simulink model "hard_threshold_fixed_multichannel"  (R2019b)
settings: Solver=VariableStepAuto  StartTime=0.0  StopTime=10  RelTol=1e-3
libraries: simulink x33, dspswit3 x1
settings Model: Creator=sbuccelli  LastModifiedBy=sbuccelli

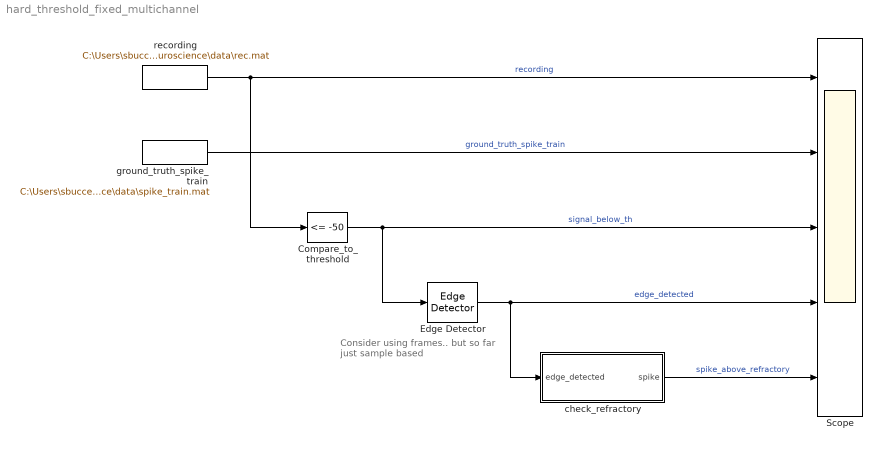
== system hard_threshold_fixed_multichannel ==
  note: Consider using frames..
      | but so far just sample based
  Compare_to_threshold : simulink/Logic and Bit Operations/Compare To Constant  relop=<=  const=-50  OutDataTypeStr=boolean
  Edge Detector : dspswit3/Edge Detector
      settings: SourceProductName=DSP System Toolbox  SourceProductBaseCode=DS
  Scope : Scope  NumInputPorts=5
  check_refractory : Subsystem
  ground_truth_spike_train : FromFile  FileName=C:\Users\sbuccelli\Documents\GitHub\closed-loop-neuroscience\data\spike_train.mat  SampleTime=1/32e3
  recording : FromFile  FileName=C:\Users\sbuccelli\Documents\GitHub\closed-loop-neuroscience\data\rec.mat  SampleTime=1/32e3
  wires:
  recording/1 -> Compare_to_threshold/1, Scope/1  "recording"
  ground_truth_spike_train/1 -> Scope/2  "ground_truth_spike_train"
  Compare_to_threshold/1 -> Edge Detector/1, Scope/3  "signal_below_th"
  Edge Detector/1 -> check_refractory/1(edge_detected), Scope/4  "edge_detected"
  check_refractory/1(spike) -> Scope/5  "spike_above_refractory"

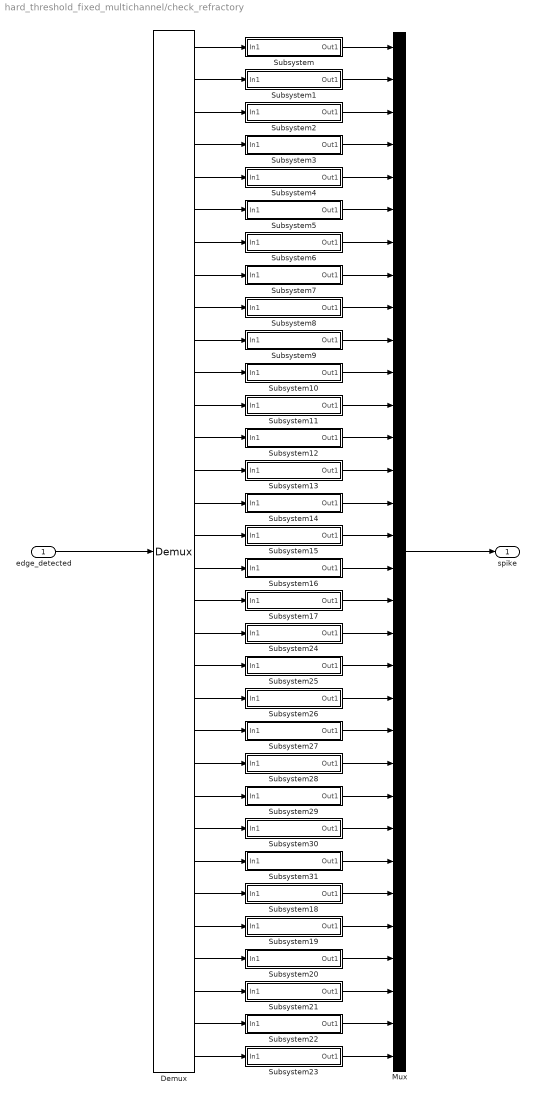
== system hard_threshold_fixed_multichannel/check_refractory ==
  edge_detected : Inport
  Demux : Demux  Outputs=32
  Mux : Mux  Inputs=32
  Subsystem : Subsystem
  Subsystem1 : Subsystem
  Subsystem10 : Subsystem
  Subsystem11 : Subsystem
  Subsystem12 : Subsystem
  Subsystem13 : Subsystem
  Subsystem14 : Subsystem
  Subsystem15 : Subsystem
  Subsystem16 : Subsystem
  Subsystem17 : Subsystem
  Subsystem18 : Subsystem
  Subsystem19 : Subsystem
  Subsystem2 : Subsystem
  Subsystem20 : Subsystem
  Subsystem21 : Subsystem
  Subsystem22 : Subsystem
  Subsystem23 : Subsystem
  Subsystem24 : Subsystem
  Subsystem25 : Subsystem
  Subsystem26 : Subsystem
  Subsystem27 : Subsystem
  Subsystem28 : Subsystem
  Subsystem29 : Subsystem
  Subsystem3 : Subsystem
  Subsystem30 : Subsystem
  Subsystem31 : Subsystem
  Subsystem4 : Subsystem
  Subsystem5 : Subsystem
  Subsystem6 : Subsystem
  Subsystem7 : Subsystem
  Subsystem8 : Subsystem
  Subsystem9 : Subsystem
  spike : Outport
  wires:
  edge_detected/1 -> Demux/1
  Demux/1 -> Subsystem/1(In1)
  Subsystem/1(Out1) -> Mux/1
  Mux/1 -> spike/1
  Subsystem1/1(Out1) -> Mux/2
  Demux/2 -> Subsystem1/1(In1)
  Demux/4 -> Subsystem3/1(In1)
  Subsystem3/1(Out1) -> Mux/4
  Subsystem2/1(Out1) -> Mux/3
  Demux/3 -> Subsystem2/1(In1)
  Demux/8 -> Subsystem7/1(In1)
  Demux/6 -> Subsystem5/1(In1)
  Subsystem5/1(Out1) -> Mux/6
  Demux/7 -> Subsystem6/1(In1)
  Subsystem7/1(Out1) -> Mux/8
  Subsystem4/1(Out1) -> Mux/5
  Subsystem6/1(Out1) -> Mux/7
  Demux/5 -> Subsystem4/1(In1)
  Subsystem15/1(Out1) -> Mux/16
  Demux/16 -> Subsystem15/1(In1)
  Subsystem12/1(Out1) -> Mux/13
  Demux/13 -> Subsystem12/1(In1)
  Demux/14 -> Subsystem13/1(In1)
  Demux/15 -> Subsystem14/1(In1)
  Subsystem14/1(Out1) -> Mux/15
  Demux/12 -> Subsystem11/1(In1)
  Demux/10 -> Subsystem9/1(In1)
  Subsystem13/1(Out1) -> Mux/14
  Subsystem9/1(Out1) -> Mux/10
  Demux/11 -> Subsystem10/1(In1)
  Subsystem11/1(Out1) -> Mux/12
  Subsystem8/1(Out1) -> Mux/9
  Subsystem10/1(Out1) -> Mux/11
  Demux/9 -> Subsystem8/1(In1)
  Subsystem23/1(Out1) -> Mux/32
  Subsystem21/1(Out1) -> Mux/30
  Subsystem22/1(Out1) -> Mux/31
  Subsystem20/1(Out1) -> Mux/29
  Demux/29 -> Subsystem20/1(In1)
  Subsystem29/1(Out1) -> Mux/24
  Demux/24 -> Subsystem29/1(In1)
  Subsystem26/1(Out1) -> Mux/21
  Demux/21 -> Subsystem26/1(In1)
  Demux/26 -> Subsystem31/1(In1)
  Demux/22 -> Subsystem27/1(In1)
  Demux/23 -> Subsystem28/1(In1)
  Subsystem27/1(Out1) -> Mux/22
  Demux/27 -> Subsystem18/1(In1)
  Demux/32 -> Subsystem23/1(In1)
  Subsystem19/1(Out1) -> Mux/28
  Subsystem18/1(Out1) -> Mux/27
  Subsystem31/1(Out1) -> Mux/26
  Subsystem28/1(Out1) -> Mux/23
  Demux/20 -> Subsystem25/1(In1)
  Subsystem30/1(Out1) -> Mux/25
  Demux/30 -> Subsystem21/1(In1)
  Demux/18 -> Subsystem17/1(In1)
  Subsystem17/1(Out1) -> Mux/18
  Demux/19 -> Subsystem24/1(In1)
  Demux/28 -> Subsystem19/1(In1)
  Subsystem25/1(Out1) -> Mux/20
  Subsystem16/1(Out1) -> Mux/17
  Subsystem24/1(Out1) -> Mux/19
  Demux/25 -> Subsystem30/1(In1)
  Demux/17 -> Subsystem16/1(In1)
  Demux/31 -> Subsystem22/1(In1)

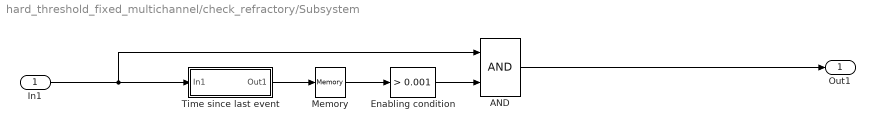
== system hard_threshold_fixed_multichannel/check_refractory/Subsystem ==
  In1 : Inport
  AND : Logic  IconShape=distinctive  AllPortsSameDT=off  OutDataTypeStr=boolean
  Enabling condition : simulink/Logic and Bit Operations/Compare To Constant  relop=>  const=0.001  OutDataTypeStr=boolean
  Memory : Memory  InheritSampleTime=on
  "Time since last event " : Subsystem
  Out1 : Outport
  wires:
  In1/1 -> AND/1, "Time since last event "/1(In1)
  Memory/1 -> Enabling condition/1
  Enabling condition/1 -> AND/2
  AND/1 -> Out1/1
  "Time since last event "/1(Out1) -> Memory/1

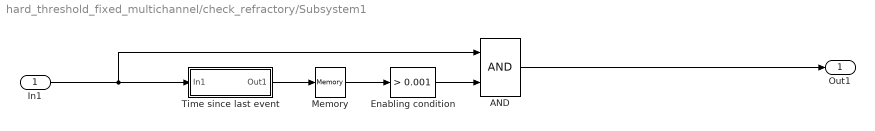
== system hard_threshold_fixed_multichannel/check_refractory/Subsystem1 ==
  In1 : Inport
  AND : Logic  IconShape=distinctive  AllPortsSameDT=off  OutDataTypeStr=boolean
  Enabling condition : simulink/Logic and Bit Operations/Compare To Constant  relop=>  const=0.001  OutDataTypeStr=boolean
  Memory : Memory  InheritSampleTime=on
  "Time since last event " : Subsystem
  Out1 : Outport
  wires:
  In1/1 -> AND/1, "Time since last event "/1(In1)
  Memory/1 -> Enabling condition/1
  Enabling condition/1 -> AND/2
  AND/1 -> Out1/1
  "Time since last event "/1(Out1) -> Memory/1

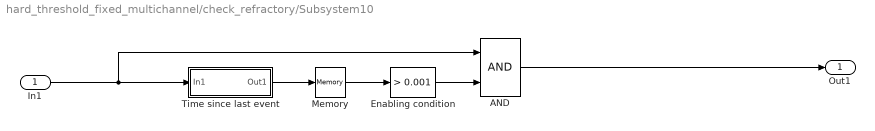
== system hard_threshold_fixed_multichannel/check_refractory/Subsystem10 ==
  In1 : Inport
  AND : Logic  IconShape=distinctive  AllPortsSameDT=off  OutDataTypeStr=boolean
  Enabling condition : simulink/Logic and Bit Operations/Compare To Constant  relop=>  const=0.001  OutDataTypeStr=boolean
  Memory : Memory  InheritSampleTime=on
  "Time since last event " : Subsystem
  Out1 : Outport
  wires:
  In1/1 -> AND/1, "Time since last event "/1(In1)
  Memory/1 -> Enabling condition/1
  Enabling condition/1 -> AND/2
  AND/1 -> Out1/1
  "Time since last event "/1(Out1) -> Memory/1

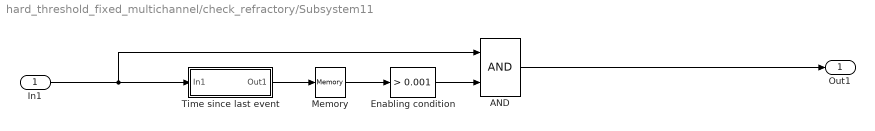
== system hard_threshold_fixed_multichannel/check_refractory/Subsystem11 ==
  In1 : Inport
  AND : Logic  IconShape=distinctive  AllPortsSameDT=off  OutDataTypeStr=boolean
  Enabling condition : simulink/Logic and Bit Operations/Compare To Constant  relop=>  const=0.001  OutDataTypeStr=boolean
  Memory : Memory  InheritSampleTime=on
  "Time since last event " : Subsystem
  Out1 : Outport
  wires:
  In1/1 -> AND/1, "Time since last event "/1(In1)
  Memory/1 -> Enabling condition/1
  Enabling condition/1 -> AND/2
  AND/1 -> Out1/1
  "Time since last event "/1(Out1) -> Memory/1

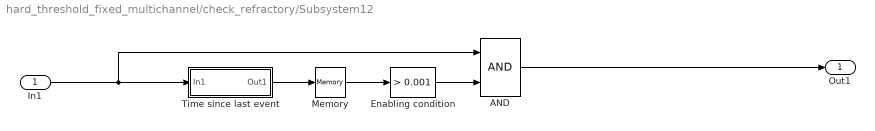
== system hard_threshold_fixed_multichannel/check_refractory/Subsystem12 ==
  In1 : Inport
  AND : Logic  IconShape=distinctive  AllPortsSameDT=off  OutDataTypeStr=boolean
  Enabling condition : simulink/Logic and Bit Operations/Compare To Constant  relop=>  const=0.001  OutDataTypeStr=boolean
  Memory : Memory  InheritSampleTime=on
  "Time since last event " : Subsystem
  Out1 : Outport
  wires:
  In1/1 -> AND/1, "Time since last event "/1(In1)
  Memory/1 -> Enabling condition/1
  Enabling condition/1 -> AND/2
  AND/1 -> Out1/1
  "Time since last event "/1(Out1) -> Memory/1

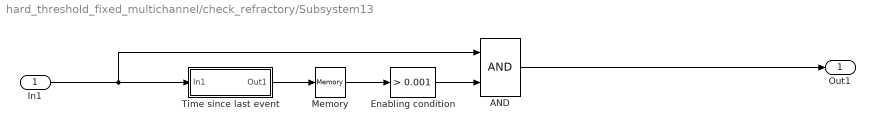
== system hard_threshold_fixed_multichannel/check_refractory/Subsystem13 ==
  In1 : Inport
  AND : Logic  IconShape=distinctive  AllPortsSameDT=off  OutDataTypeStr=boolean
  Enabling condition : simulink/Logic and Bit Operations/Compare To Constant  relop=>  const=0.001  OutDataTypeStr=boolean
  Memory : Memory  InheritSampleTime=on
  "Time since last event " : Subsystem
  Out1 : Outport
  wires:
  In1/1 -> AND/1, "Time since last event "/1(In1)
  Memory/1 -> Enabling condition/1
  Enabling condition/1 -> AND/2
  AND/1 -> Out1/1
  "Time since last event "/1(Out1) -> Memory/1

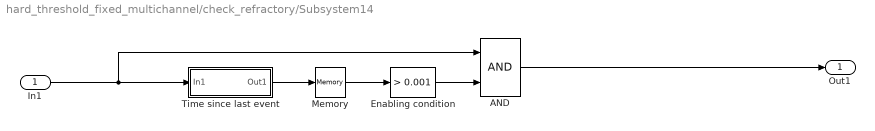
== system hard_threshold_fixed_multichannel/check_refractory/Subsystem14 ==
  In1 : Inport
  AND : Logic  IconShape=distinctive  AllPortsSameDT=off  OutDataTypeStr=boolean
  Enabling condition : simulink/Logic and Bit Operations/Compare To Constant  relop=>  const=0.001  OutDataTypeStr=boolean
  Memory : Memory  InheritSampleTime=on
  "Time since last event " : Subsystem
  Out1 : Outport
  wires:
  In1/1 -> AND/1, "Time since last event "/1(In1)
  Memory/1 -> Enabling condition/1
  Enabling condition/1 -> AND/2
  AND/1 -> Out1/1
  "Time since last event "/1(Out1) -> Memory/1

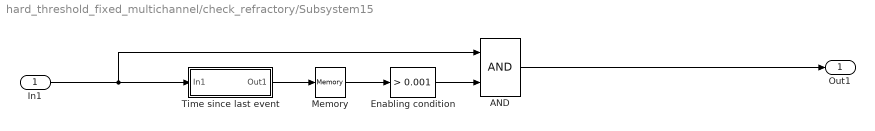
== system hard_threshold_fixed_multichannel/check_refractory/Subsystem15 ==
  In1 : Inport
  AND : Logic  IconShape=distinctive  AllPortsSameDT=off  OutDataTypeStr=boolean
  Enabling condition : simulink/Logic and Bit Operations/Compare To Constant  relop=>  const=0.001  OutDataTypeStr=boolean
  Memory : Memory  InheritSampleTime=on
  "Time since last event " : Subsystem
  Out1 : Outport
  wires:
  In1/1 -> AND/1, "Time since last event "/1(In1)
  Memory/1 -> Enabling condition/1
  Enabling condition/1 -> AND/2
  AND/1 -> Out1/1
  "Time since last event "/1(Out1) -> Memory/1

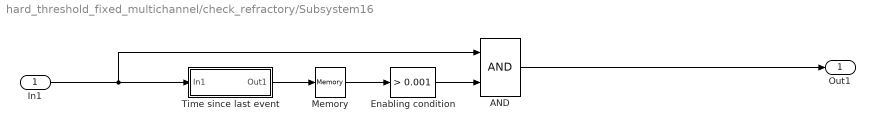
== system hard_threshold_fixed_multichannel/check_refractory/Subsystem16 ==
  In1 : Inport
  AND : Logic  IconShape=distinctive  AllPortsSameDT=off  OutDataTypeStr=boolean
  Enabling condition : simulink/Logic and Bit Operations/Compare To Constant  relop=>  const=0.001  OutDataTypeStr=boolean
  Memory : Memory  InheritSampleTime=on
  "Time since last event " : Subsystem
  Out1 : Outport
  wires:
  In1/1 -> AND/1, "Time since last event "/1(In1)
  Memory/1 -> Enabling condition/1
  Enabling condition/1 -> AND/2
  AND/1 -> Out1/1
  "Time since last event "/1(Out1) -> Memory/1

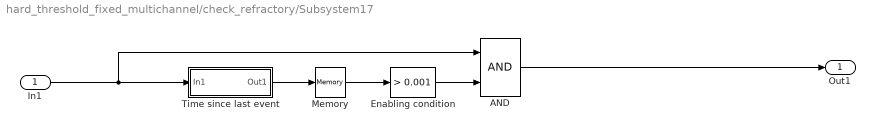
== system hard_threshold_fixed_multichannel/check_refractory/Subsystem17 ==
  In1 : Inport
  AND : Logic  IconShape=distinctive  AllPortsSameDT=off  OutDataTypeStr=boolean
  Enabling condition : simulink/Logic and Bit Operations/Compare To Constant  relop=>  const=0.001  OutDataTypeStr=boolean
  Memory : Memory  InheritSampleTime=on
  "Time since last event " : Subsystem
  Out1 : Outport
  wires:
  In1/1 -> AND/1, "Time since last event "/1(In1)
  Memory/1 -> Enabling condition/1
  Enabling condition/1 -> AND/2
  AND/1 -> Out1/1
  "Time since last event "/1(Out1) -> Memory/1

== system hard_threshold_fixed_multichannel/check_refractory/Subsystem18 ==
  In1 : Inport
  AND : Logic  IconShape=distinctive  AllPortsSameDT=off  OutDataTypeStr=boolean
  Enabling condition : simulink/Logic and Bit Operations/Compare To Constant  relop=>  const=0.001  OutDataTypeStr=boolean
  Memory : Memory  InheritSampleTime=on
  "Time since last event " : Subsystem
  Out1 : Outport
  wires:
  In1/1 -> AND/1, "Time since last event "/1(In1)
  Memory/1 -> Enabling condition/1
  Enabling condition/1 -> AND/2
  AND/1 -> Out1/1
  "Time since last event "/1(Out1) -> Memory/1

== system hard_threshold_fixed_multichannel/check_refractory/Subsystem19 ==
  In1 : Inport
  AND : Logic  IconShape=distinctive  AllPortsSameDT=off  OutDataTypeStr=boolean
  Enabling condition : simulink/Logic and Bit Operations/Compare To Constant  relop=>  const=0.001  OutDataTypeStr=boolean
  Memory : Memory  InheritSampleTime=on
  "Time since last event " : Subsystem
  Out1 : Outport
  wires:
  In1/1 -> AND/1, "Time since last event "/1(In1)
  Memory/1 -> Enabling condition/1
  Enabling condition/1 -> AND/2
  AND/1 -> Out1/1
  "Time since last event "/1(Out1) -> Memory/1

== system hard_threshold_fixed_multichannel/check_refractory/Subsystem2 ==
  In1 : Inport
  AND : Logic  IconShape=distinctive  AllPortsSameDT=off  OutDataTypeStr=boolean
  Enabling condition : simulink/Logic and Bit Operations/Compare To Constant  relop=>  const=0.001  OutDataTypeStr=boolean
  Memory : Memory  InheritSampleTime=on
  "Time since last event " : Subsystem
  Out1 : Outport
  wires:
  In1/1 -> AND/1, "Time since last event "/1(In1)
  Memory/1 -> Enabling condition/1
  Enabling condition/1 -> AND/2
  AND/1 -> Out1/1
  "Time since last event "/1(Out1) -> Memory/1

== system hard_threshold_fixed_multichannel/check_refractory/Subsystem20 ==
  In1 : Inport
  AND : Logic  IconShape=distinctive  AllPortsSameDT=off  OutDataTypeStr=boolean
  Enabling condition : simulink/Logic and Bit Operations/Compare To Constant  relop=>  const=0.001  OutDataTypeStr=boolean
  Memory : Memory  InheritSampleTime=on
  "Time since last event " : Subsystem
  Out1 : Outport
  wires:
  In1/1 -> AND/1, "Time since last event "/1(In1)
  Memory/1 -> Enabling condition/1
  Enabling condition/1 -> AND/2
  AND/1 -> Out1/1
  "Time since last event "/1(Out1) -> Memory/1

== system hard_threshold_fixed_multichannel/check_refractory/Subsystem21 ==
  In1 : Inport
  AND : Logic  IconShape=distinctive  AllPortsSameDT=off  OutDataTypeStr=boolean
  Enabling condition : simulink/Logic and Bit Operations/Compare To Constant  relop=>  const=0.001  OutDataTypeStr=boolean
  Memory : Memory  InheritSampleTime=on
  "Time since last event " : Subsystem
  Out1 : Outport
  wires:
  In1/1 -> AND/1, "Time since last event "/1(In1)
  Memory/1 -> Enabling condition/1
  Enabling condition/1 -> AND/2
  AND/1 -> Out1/1
  "Time since last event "/1(Out1) -> Memory/1

== system hard_threshold_fixed_multichannel/check_refractory/Subsystem22 ==
  In1 : Inport
  AND : Logic  IconShape=distinctive  AllPortsSameDT=off  OutDataTypeStr=boolean
  Enabling condition : simulink/Logic and Bit Operations/Compare To Constant  relop=>  const=0.001  OutDataTypeStr=boolean
  Memory : Memory  InheritSampleTime=on
  "Time since last event " : Subsystem
  Out1 : Outport
  wires:
  In1/1 -> AND/1, "Time since last event "/1(In1)
  Memory/1 -> Enabling condition/1
  Enabling condition/1 -> AND/2
  AND/1 -> Out1/1
  "Time since last event "/1(Out1) -> Memory/1

== system hard_threshold_fixed_multichannel/check_refractory/Subsystem23 ==
  In1 : Inport
  AND : Logic  IconShape=distinctive  AllPortsSameDT=off  OutDataTypeStr=boolean
  Enabling condition : simulink/Logic and Bit Operations/Compare To Constant  relop=>  const=0.001  OutDataTypeStr=boolean
  Memory : Memory  InheritSampleTime=on
  "Time since last event " : Subsystem
  Out1 : Outport
  wires:
  In1/1 -> AND/1, "Time since last event "/1(In1)
  Memory/1 -> Enabling condition/1
  Enabling condition/1 -> AND/2
  AND/1 -> Out1/1
  "Time since last event "/1(Out1) -> Memory/1

== system hard_threshold_fixed_multichannel/check_refractory/Subsystem24 ==
  In1 : Inport
  AND : Logic  IconShape=distinctive  AllPortsSameDT=off  OutDataTypeStr=boolean
  Enabling condition : simulink/Logic and Bit Operations/Compare To Constant  relop=>  const=0.001  OutDataTypeStr=boolean
  Memory : Memory  InheritSampleTime=on
  "Time since last event " : Subsystem
  Out1 : Outport
  wires:
  In1/1 -> AND/1, "Time since last event "/1(In1)
  Memory/1 -> Enabling condition/1
  Enabling condition/1 -> AND/2
  AND/1 -> Out1/1
  "Time since last event "/1(Out1) -> Memory/1

== system hard_threshold_fixed_multichannel/check_refractory/Subsystem25 ==
  In1 : Inport
  AND : Logic  IconShape=distinctive  AllPortsSameDT=off  OutDataTypeStr=boolean
  Enabling condition : simulink/Logic and Bit Operations/Compare To Constant  relop=>  const=0.001  OutDataTypeStr=boolean
  Memory : Memory  InheritSampleTime=on
  "Time since last event " : Subsystem
  Out1 : Outport
  wires:
  In1/1 -> AND/1, "Time since last event "/1(In1)
  Memory/1 -> Enabling condition/1
  Enabling condition/1 -> AND/2
  AND/1 -> Out1/1
  "Time since last event "/1(Out1) -> Memory/1

== system hard_threshold_fixed_multichannel/check_refractory/Subsystem26 ==
  In1 : Inport
  AND : Logic  IconShape=distinctive  AllPortsSameDT=off  OutDataTypeStr=boolean
  Enabling condition : simulink/Logic and Bit Operations/Compare To Constant  relop=>  const=0.001  OutDataTypeStr=boolean
  Memory : Memory  InheritSampleTime=on
  "Time since last event " : Subsystem
  Out1 : Outport
  wires:
  In1/1 -> AND/1, "Time since last event "/1(In1)
  Memory/1 -> Enabling condition/1
  Enabling condition/1 -> AND/2
  AND/1 -> Out1/1
  "Time since last event "/1(Out1) -> Memory/1

== system hard_threshold_fixed_multichannel/check_refractory/Subsystem27 ==
  In1 : Inport
  AND : Logic  IconShape=distinctive  AllPortsSameDT=off  OutDataTypeStr=boolean
  Enabling condition : simulink/Logic and Bit Operations/Compare To Constant  relop=>  const=0.001  OutDataTypeStr=boolean
  Memory : Memory  InheritSampleTime=on
  "Time since last event " : Subsystem
  Out1 : Outport
  wires:
  In1/1 -> AND/1, "Time since last event "/1(In1)
  Memory/1 -> Enabling condition/1
  Enabling condition/1 -> AND/2
  AND/1 -> Out1/1
  "Time since last event "/1(Out1) -> Memory/1

== system hard_threshold_fixed_multichannel/check_refractory/Subsystem28 ==
  In1 : Inport
  AND : Logic  IconShape=distinctive  AllPortsSameDT=off  OutDataTypeStr=boolean
  Enabling condition : simulink/Logic and Bit Operations/Compare To Constant  relop=>  const=0.001  OutDataTypeStr=boolean
  Memory : Memory  InheritSampleTime=on
  "Time since last event " : Subsystem
  Out1 : Outport
  wires:
  In1/1 -> AND/1, "Time since last event "/1(In1)
  Memory/1 -> Enabling condition/1
  Enabling condition/1 -> AND/2
  AND/1 -> Out1/1
  "Time since last event "/1(Out1) -> Memory/1

== system hard_threshold_fixed_multichannel/check_refractory/Subsystem29 ==
  In1 : Inport
  AND : Logic  IconShape=distinctive  AllPortsSameDT=off  OutDataTypeStr=boolean
  Enabling condition : simulink/Logic and Bit Operations/Compare To Constant  relop=>  const=0.001  OutDataTypeStr=boolean
  Memory : Memory  InheritSampleTime=on
  "Time since last event " : Subsystem
  Out1 : Outport
  wires:
  In1/1 -> AND/1, "Time since last event "/1(In1)
  Memory/1 -> Enabling condition/1
  Enabling condition/1 -> AND/2
  AND/1 -> Out1/1
  "Time since last event "/1(Out1) -> Memory/1

== system hard_threshold_fixed_multichannel/check_refractory/Subsystem3 ==
  In1 : Inport
  AND : Logic  IconShape=distinctive  AllPortsSameDT=off  OutDataTypeStr=boolean
  Enabling condition : simulink/Logic and Bit Operations/Compare To Constant  relop=>  const=0.001  OutDataTypeStr=boolean
  Memory : Memory  InheritSampleTime=on
  "Time since last event " : Subsystem
  Out1 : Outport
  wires:
  In1/1 -> AND/1, "Time since last event "/1(In1)
  Memory/1 -> Enabling condition/1
  Enabling condition/1 -> AND/2
  AND/1 -> Out1/1
  "Time since last event "/1(Out1) -> Memory/1

== system hard_threshold_fixed_multichannel/check_refractory/Subsystem30 ==
  In1 : Inport
  AND : Logic  IconShape=distinctive  AllPortsSameDT=off  OutDataTypeStr=boolean
  Enabling condition : simulink/Logic and Bit Operations/Compare To Constant  relop=>  const=0.001  OutDataTypeStr=boolean
  Memory : Memory  InheritSampleTime=on
  "Time since last event " : Subsystem
  Out1 : Outport
  wires:
  In1/1 -> AND/1, "Time since last event "/1(In1)
  Memory/1 -> Enabling condition/1
  Enabling condition/1 -> AND/2
  AND/1 -> Out1/1
  "Time since last event "/1(Out1) -> Memory/1

== system hard_threshold_fixed_multichannel/check_refractory/Subsystem31 ==
  In1 : Inport
  AND : Logic  IconShape=distinctive  AllPortsSameDT=off  OutDataTypeStr=boolean
  Enabling condition : simulink/Logic and Bit Operations/Compare To Constant  relop=>  const=0.001  OutDataTypeStr=boolean
  Memory : Memory  InheritSampleTime=on
  "Time since last event " : Subsystem
  Out1 : Outport
  wires:
  In1/1 -> AND/1, "Time since last event "/1(In1)
  Memory/1 -> Enabling condition/1
  Enabling condition/1 -> AND/2
  AND/1 -> Out1/1
  "Time since last event "/1(Out1) -> Memory/1

== system hard_threshold_fixed_multichannel/check_refractory/Subsystem4 ==
  In1 : Inport
  AND : Logic  IconShape=distinctive  AllPortsSameDT=off  OutDataTypeStr=boolean
  Enabling condition : simulink/Logic and Bit Operations/Compare To Constant  relop=>  const=0.001  OutDataTypeStr=boolean
  Memory : Memory  InheritSampleTime=on
  "Time since last event " : Subsystem
  Out1 : Outport
  wires:
  In1/1 -> AND/1, "Time since last event "/1(In1)
  Memory/1 -> Enabling condition/1
  Enabling condition/1 -> AND/2
  AND/1 -> Out1/1
  "Time since last event "/1(Out1) -> Memory/1

== system hard_threshold_fixed_multichannel/check_refractory/Subsystem5 ==
  In1 : Inport
  AND : Logic  IconShape=distinctive  AllPortsSameDT=off  OutDataTypeStr=boolean
  Enabling condition : simulink/Logic and Bit Operations/Compare To Constant  relop=>  const=0.001  OutDataTypeStr=boolean
  Memory : Memory  InheritSampleTime=on
  "Time since last event " : Subsystem
  Out1 : Outport
  wires:
  In1/1 -> AND/1, "Time since last event "/1(In1)
  Memory/1 -> Enabling condition/1
  Enabling condition/1 -> AND/2
  AND/1 -> Out1/1
  "Time since last event "/1(Out1) -> Memory/1

== system hard_threshold_fixed_multichannel/check_refractory/Subsystem6 ==
  In1 : Inport
  AND : Logic  IconShape=distinctive  AllPortsSameDT=off  OutDataTypeStr=boolean
  Enabling condition : simulink/Logic and Bit Operations/Compare To Constant  relop=>  const=0.001  OutDataTypeStr=boolean
  Memory : Memory  InheritSampleTime=on
  "Time since last event " : Subsystem
  Out1 : Outport
  wires:
  In1/1 -> AND/1, "Time since last event "/1(In1)
  Memory/1 -> Enabling condition/1
  Enabling condition/1 -> AND/2
  AND/1 -> Out1/1
  "Time since last event "/1(Out1) -> Memory/1

== system hard_threshold_fixed_multichannel/check_refractory/Subsystem7 ==
  In1 : Inport
  AND : Logic  IconShape=distinctive  AllPortsSameDT=off  OutDataTypeStr=boolean
  Enabling condition : simulink/Logic and Bit Operations/Compare To Constant  relop=>  const=0.001  OutDataTypeStr=boolean
  Memory : Memory  InheritSampleTime=on
  "Time since last event " : Subsystem
  Out1 : Outport
  wires:
  In1/1 -> AND/1, "Time since last event "/1(In1)
  Memory/1 -> Enabling condition/1
  Enabling condition/1 -> AND/2
  AND/1 -> Out1/1
  "Time since last event "/1(Out1) -> Memory/1

== system hard_threshold_fixed_multichannel/check_refractory/Subsystem8 ==
  In1 : Inport
  AND : Logic  IconShape=distinctive  AllPortsSameDT=off  OutDataTypeStr=boolean
  Enabling condition : simulink/Logic and Bit Operations/Compare To Constant  relop=>  const=0.001  OutDataTypeStr=boolean
  Memory : Memory  InheritSampleTime=on
  "Time since last event " : Subsystem
  Out1 : Outport
  wires:
  In1/1 -> AND/1, "Time since last event "/1(In1)
  Memory/1 -> Enabling condition/1
  Enabling condition/1 -> AND/2
  AND/1 -> Out1/1
  "Time since last event "/1(Out1) -> Memory/1

== system hard_threshold_fixed_multichannel/check_refractory/Subsystem9 ==
  In1 : Inport
  AND : Logic  IconShape=distinctive  AllPortsSameDT=off  OutDataTypeStr=boolean
  Enabling condition : simulink/Logic and Bit Operations/Compare To Constant  relop=>  const=0.001  OutDataTypeStr=boolean
  Memory : Memory  InheritSampleTime=on
  "Time since last event " : Subsystem
  Out1 : Outport
  wires:
  In1/1 -> AND/1, "Time since last event "/1(In1)
  Memory/1 -> Enabling condition/1
  Enabling condition/1 -> AND/2
  AND/1 -> Out1/1
  "Time since last event "/1(Out1) -> Memory/1

== system hard_threshold_fixed_multichannel/check_refractory/Subsystem/Time since last event  ==
  In1 : Inport
  Digital Clock : DigitalClock  SampleTime=1/32e3
  Sum : Sum  Inputs=|-+
  Triggered Subsystem : Subsystem  TreatAsAtomicUnit=on
  Out1 : Outport
  wires:
  Digital Clock/1 -> Sum/2, Triggered Subsystem/1(In1)
  Triggered Subsystem/1(Out1) -> Sum/1
  In1/1 -> Triggered Subsystem/Trigger
  Sum/1 -> Out1/1

== system hard_threshold_fixed_multichannel/check_refractory/Subsystem1/Time since last event  ==
  In1 : Inport
  Digital Clock : DigitalClock  SampleTime=1/32e3
  Sum : Sum  Inputs=|-+
  Triggered Subsystem : Subsystem  TreatAsAtomicUnit=on
  Out1 : Outport
  wires:
  Digital Clock/1 -> Sum/2, Triggered Subsystem/1(In1)
  Triggered Subsystem/1(Out1) -> Sum/1
  In1/1 -> Triggered Subsystem/Trigger
  Sum/1 -> Out1/1

== system hard_threshold_fixed_multichannel/check_refractory/Subsystem10/Time since last event  ==
  In1 : Inport
  Digital Clock : DigitalClock  SampleTime=1/32e3
  Sum : Sum  Inputs=|-+
  Triggered Subsystem : Subsystem  TreatAsAtomicUnit=on
  Out1 : Outport
  wires:
  Digital Clock/1 -> Sum/2, Triggered Subsystem/1(In1)
  Triggered Subsystem/1(Out1) -> Sum/1
  In1/1 -> Triggered Subsystem/Trigger
  Sum/1 -> Out1/1

== system hard_threshold_fixed_multichannel/check_refractory/Subsystem11/Time since last event  ==
  In1 : Inport
  Digital Clock : DigitalClock  SampleTime=1/32e3
  Sum : Sum  Inputs=|-+
  Triggered Subsystem : Subsystem  TreatAsAtomicUnit=on
  Out1 : Outport
  wires:
  Digital Clock/1 -> Sum/2, Triggered Subsystem/1(In1)
  Triggered Subsystem/1(Out1) -> Sum/1
  In1/1 -> Triggered Subsystem/Trigger
  Sum/1 -> Out1/1

== system hard_threshold_fixed_multichannel/check_refractory/Subsystem12/Time since last event  ==
  In1 : Inport
  Digital Clock : DigitalClock  SampleTime=1/32e3
  Sum : Sum  Inputs=|-+
  Triggered Subsystem : Subsystem  TreatAsAtomicUnit=on
  Out1 : Outport
  wires:
  Digital Clock/1 -> Sum/2, Triggered Subsystem/1(In1)
  Triggered Subsystem/1(Out1) -> Sum/1
  In1/1 -> Triggered Subsystem/Trigger
  Sum/1 -> Out1/1

== system hard_threshold_fixed_multichannel/check_refractory/Subsystem13/Time since last event  ==
  In1 : Inport
  Digital Clock : DigitalClock  SampleTime=1/32e3
  Sum : Sum  Inputs=|-+
  Triggered Subsystem : Subsystem  TreatAsAtomicUnit=on
  Out1 : Outport
  wires:
  Digital Clock/1 -> Sum/2, Triggered Subsystem/1(In1)
  Triggered Subsystem/1(Out1) -> Sum/1
  In1/1 -> Triggered Subsystem/Trigger
  Sum/1 -> Out1/1

== system hard_threshold_fixed_multichannel/check_refractory/Subsystem14/Time since last event  ==
  In1 : Inport
  Digital Clock : DigitalClock  SampleTime=1/32e3
  Sum : Sum  Inputs=|-+
  Triggered Subsystem : Subsystem  TreatAsAtomicUnit=on
  Out1 : Outport
  wires:
  Digital Clock/1 -> Sum/2, Triggered Subsystem/1(In1)
  Triggered Subsystem/1(Out1) -> Sum/1
  In1/1 -> Triggered Subsystem/Trigger
  Sum/1 -> Out1/1

== system hard_threshold_fixed_multichannel/check_refractory/Subsystem15/Time since last event  ==
  In1 : Inport
  Digital Clock : DigitalClock  SampleTime=1/32e3
  Sum : Sum  Inputs=|-+
  Triggered Subsystem : Subsystem  TreatAsAtomicUnit=on
  Out1 : Outport
  wires:
  Digital Clock/1 -> Sum/2, Triggered Subsystem/1(In1)
  Triggered Subsystem/1(Out1) -> Sum/1
  In1/1 -> Triggered Subsystem/Trigger
  Sum/1 -> Out1/1

== system hard_threshold_fixed_multichannel/check_refractory/Subsystem16/Time since last event  ==
  In1 : Inport
  Digital Clock : DigitalClock  SampleTime=1/32e3
  Sum : Sum  Inputs=|-+
  Triggered Subsystem : Subsystem  TreatAsAtomicUnit=on
  Out1 : Outport
  wires:
  Digital Clock/1 -> Sum/2, Triggered Subsystem/1(In1)
  Triggered Subsystem/1(Out1) -> Sum/1
  In1/1 -> Triggered Subsystem/Trigger
  Sum/1 -> Out1/1

== system hard_threshold_fixed_multichannel/check_refractory/Subsystem17/Time since last event  ==
  In1 : Inport
  Digital Clock : DigitalClock  SampleTime=1/32e3
  Sum : Sum  Inputs=|-+
  Triggered Subsystem : Subsystem  TreatAsAtomicUnit=on
  Out1 : Outport
  wires:
  Digital Clock/1 -> Sum/2, Triggered Subsystem/1(In1)
  Triggered Subsystem/1(Out1) -> Sum/1
  In1/1 -> Triggered Subsystem/Trigger
  Sum/1 -> Out1/1

== system hard_threshold_fixed_multichannel/check_refractory/Subsystem18/Time since last event  ==
  In1 : Inport
  Digital Clock : DigitalClock  SampleTime=1/32e3
  Sum : Sum  Inputs=|-+
  Triggered Subsystem : Subsystem  TreatAsAtomicUnit=on
  Out1 : Outport
  wires:
  Digital Clock/1 -> Sum/2, Triggered Subsystem/1(In1)
  Triggered Subsystem/1(Out1) -> Sum/1
  In1/1 -> Triggered Subsystem/Trigger
  Sum/1 -> Out1/1

== system hard_threshold_fixed_multichannel/check_refractory/Subsystem19/Time since last event  ==
  In1 : Inport
  Digital Clock : DigitalClock  SampleTime=1/32e3
  Sum : Sum  Inputs=|-+
  Triggered Subsystem : Subsystem  TreatAsAtomicUnit=on
  Out1 : Outport
  wires:
  Digital Clock/1 -> Sum/2, Triggered Subsystem/1(In1)
  Triggered Subsystem/1(Out1) -> Sum/1
  In1/1 -> Triggered Subsystem/Trigger
  Sum/1 -> Out1/1

== system hard_threshold_fixed_multichannel/check_refractory/Subsystem2/Time since last event  ==
  In1 : Inport
  Digital Clock : DigitalClock  SampleTime=1/32e3
  Sum : Sum  Inputs=|-+
  Triggered Subsystem : Subsystem  TreatAsAtomicUnit=on
  Out1 : Outport
  wires:
  Digital Clock/1 -> Sum/2, Triggered Subsystem/1(In1)
  Triggered Subsystem/1(Out1) -> Sum/1
  In1/1 -> Triggered Subsystem/Trigger
  Sum/1 -> Out1/1

== system hard_threshold_fixed_multichannel/check_refractory/Subsystem20/Time since last event  ==
  In1 : Inport
  Digital Clock : DigitalClock  SampleTime=1/32e3
  Sum : Sum  Inputs=|-+
  Triggered Subsystem : Subsystem  TreatAsAtomicUnit=on
  Out1 : Outport
  wires:
  Digital Clock/1 -> Sum/2, Triggered Subsystem/1(In1)
  Triggered Subsystem/1(Out1) -> Sum/1
  In1/1 -> Triggered Subsystem/Trigger
  Sum/1 -> Out1/1

== system hard_threshold_fixed_multichannel/check_refractory/Subsystem21/Time since last event  ==
  In1 : Inport
  Digital Clock : DigitalClock  SampleTime=1/32e3
  Sum : Sum  Inputs=|-+
  Triggered Subsystem : Subsystem  TreatAsAtomicUnit=on
  Out1 : Outport
  wires:
  Digital Clock/1 -> Sum/2, Triggered Subsystem/1(In1)
  Triggered Subsystem/1(Out1) -> Sum/1
  In1/1 -> Triggered Subsystem/Trigger
  Sum/1 -> Out1/1

== system hard_threshold_fixed_multichannel/check_refractory/Subsystem22/Time since last event  ==
  In1 : Inport
  Digital Clock : DigitalClock  SampleTime=1/32e3
  Sum : Sum  Inputs=|-+
  Triggered Subsystem : Subsystem  TreatAsAtomicUnit=on
  Out1 : Outport
  wires:
  Digital Clock/1 -> Sum/2, Triggered Subsystem/1(In1)
  Triggered Subsystem/1(Out1) -> Sum/1
  In1/1 -> Triggered Subsystem/Trigger
  Sum/1 -> Out1/1

== system hard_threshold_fixed_multichannel/check_refractory/Subsystem23/Time since last event  ==
  In1 : Inport
  Digital Clock : DigitalClock  SampleTime=1/32e3
  Sum : Sum  Inputs=|-+
  Triggered Subsystem : Subsystem  TreatAsAtomicUnit=on
  Out1 : Outport
  wires:
  Digital Clock/1 -> Sum/2, Triggered Subsystem/1(In1)
  Triggered Subsystem/1(Out1) -> Sum/1
  In1/1 -> Triggered Subsystem/Trigger
  Sum/1 -> Out1/1

== system hard_threshold_fixed_multichannel/check_refractory/Subsystem24/Time since last event  ==
  In1 : Inport
  Digital Clock : DigitalClock  SampleTime=1/32e3
  Sum : Sum  Inputs=|-+
  Triggered Subsystem : Subsystem  TreatAsAtomicUnit=on
  Out1 : Outport
  wires:
  Digital Clock/1 -> Sum/2, Triggered Subsystem/1(In1)
  Triggered Subsystem/1(Out1) -> Sum/1
  In1/1 -> Triggered Subsystem/Trigger
  Sum/1 -> Out1/1

== system hard_threshold_fixed_multichannel/check_refractory/Subsystem25/Time since last event  ==
  In1 : Inport
  Digital Clock : DigitalClock  SampleTime=1/32e3
  Sum : Sum  Inputs=|-+
  Triggered Subsystem : Subsystem  TreatAsAtomicUnit=on
  Out1 : Outport
  wires:
  Digital Clock/1 -> Sum/2, Triggered Subsystem/1(In1)
  Triggered Subsystem/1(Out1) -> Sum/1
  In1/1 -> Triggered Subsystem/Trigger
  Sum/1 -> Out1/1

== system hard_threshold_fixed_multichannel/check_refractory/Subsystem26/Time since last event  ==
  In1 : Inport
  Digital Clock : DigitalClock  SampleTime=1/32e3
  Sum : Sum  Inputs=|-+
  Triggered Subsystem : Subsystem  TreatAsAtomicUnit=on
  Out1 : Outport
  wires:
  Digital Clock/1 -> Sum/2, Triggered Subsystem/1(In1)
  Triggered Subsystem/1(Out1) -> Sum/1
  In1/1 -> Triggered Subsystem/Trigger
  Sum/1 -> Out1/1

== system hard_threshold_fixed_multichannel/check_refractory/Subsystem27/Time since last event  ==
  In1 : Inport
  Digital Clock : DigitalClock  SampleTime=1/32e3
  Sum : Sum  Inputs=|-+
  Triggered Subsystem : Subsystem  TreatAsAtomicUnit=on
  Out1 : Outport
  wires:
  Digital Clock/1 -> Sum/2, Triggered Subsystem/1(In1)
  Triggered Subsystem/1(Out1) -> Sum/1
  In1/1 -> Triggered Subsystem/Trigger
  Sum/1 -> Out1/1

== system hard_threshold_fixed_multichannel/check_refractory/Subsystem28/Time since last event  ==
  In1 : Inport
  Digital Clock : DigitalClock  SampleTime=1/32e3
  Sum : Sum  Inputs=|-+
  Triggered Subsystem : Subsystem  TreatAsAtomicUnit=on
  Out1 : Outport
  wires:
  Digital Clock/1 -> Sum/2, Triggered Subsystem/1(In1)
  Triggered Subsystem/1(Out1) -> Sum/1
  In1/1 -> Triggered Subsystem/Trigger
  Sum/1 -> Out1/1

== system hard_threshold_fixed_multichannel/check_refractory/Subsystem29/Time since last event  ==
  In1 : Inport
  Digital Clock : DigitalClock  SampleTime=1/32e3
  Sum : Sum  Inputs=|-+
  Triggered Subsystem : Subsystem  TreatAsAtomicUnit=on
  Out1 : Outport
  wires:
  Digital Clock/1 -> Sum/2, Triggered Subsystem/1(In1)
  Triggered Subsystem/1(Out1) -> Sum/1
  In1/1 -> Triggered Subsystem/Trigger
  Sum/1 -> Out1/1

== system hard_threshold_fixed_multichannel/check_refractory/Subsystem3/Time since last event  ==
  In1 : Inport
  Digital Clock : DigitalClock  SampleTime=1/32e3
  Sum : Sum  Inputs=|-+
  Triggered Subsystem : Subsystem  TreatAsAtomicUnit=on
  Out1 : Outport
  wires:
  Digital Clock/1 -> Sum/2, Triggered Subsystem/1(In1)
  Triggered Subsystem/1(Out1) -> Sum/1
  In1/1 -> Triggered Subsystem/Trigger
  Sum/1 -> Out1/1

== system hard_threshold_fixed_multichannel/check_refractory/Subsystem30/Time since last event  ==
  In1 : Inport
  Digital Clock : DigitalClock  SampleTime=1/32e3
  Sum : Sum  Inputs=|-+
  Triggered Subsystem : Subsystem  TreatAsAtomicUnit=on
  Out1 : Outport
  wires:
  Digital Clock/1 -> Sum/2, Triggered Subsystem/1(In1)
  Triggered Subsystem/1(Out1) -> Sum/1
  In1/1 -> Triggered Subsystem/Trigger
  Sum/1 -> Out1/1

== system hard_threshold_fixed_multichannel/check_refractory/Subsystem31/Time since last event  ==
  In1 : Inport
  Digital Clock : DigitalClock  SampleTime=1/32e3
  Sum : Sum  Inputs=|-+
  Triggered Subsystem : Subsystem  TreatAsAtomicUnit=on
  Out1 : Outport
  wires:
  Digital Clock/1 -> Sum/2, Triggered Subsystem/1(In1)
  Triggered Subsystem/1(Out1) -> Sum/1
  In1/1 -> Triggered Subsystem/Trigger
  Sum/1 -> Out1/1

== system hard_threshold_fixed_multichannel/check_refractory/Subsystem4/Time since last event  ==
  In1 : Inport
  Digital Clock : DigitalClock  SampleTime=1/32e3
  Sum : Sum  Inputs=|-+
  Triggered Subsystem : Subsystem  TreatAsAtomicUnit=on
  Out1 : Outport
  wires:
  Digital Clock/1 -> Sum/2, Triggered Subsystem/1(In1)
  Triggered Subsystem/1(Out1) -> Sum/1
  In1/1 -> Triggered Subsystem/Trigger
  Sum/1 -> Out1/1

== system hard_threshold_fixed_multichannel/check_refractory/Subsystem5/Time since last event  ==
  In1 : Inport
  Digital Clock : DigitalClock  SampleTime=1/32e3
  Sum : Sum  Inputs=|-+
  Triggered Subsystem : Subsystem  TreatAsAtomicUnit=on
  Out1 : Outport
  wires:
  Digital Clock/1 -> Sum/2, Triggered Subsystem/1(In1)
  Triggered Subsystem/1(Out1) -> Sum/1
  In1/1 -> Triggered Subsystem/Trigger
  Sum/1 -> Out1/1

== system hard_threshold_fixed_multichannel/check_refractory/Subsystem6/Time since last event  ==
  In1 : Inport
  Digital Clock : DigitalClock  SampleTime=1/32e3
  Sum : Sum  Inputs=|-+
  Triggered Subsystem : Subsystem  TreatAsAtomicUnit=on
  Out1 : Outport
  wires:
  Digital Clock/1 -> Sum/2, Triggered Subsystem/1(In1)
  Triggered Subsystem/1(Out1) -> Sum/1
  In1/1 -> Triggered Subsystem/Trigger
  Sum/1 -> Out1/1

== system hard_threshold_fixed_multichannel/check_refractory/Subsystem7/Time since last event  ==
  In1 : Inport
  Digital Clock : DigitalClock  SampleTime=1/32e3
  Sum : Sum  Inputs=|-+
  Triggered Subsystem : Subsystem  TreatAsAtomicUnit=on
  Out1 : Outport
  wires:
  Digital Clock/1 -> Sum/2, Triggered Subsystem/1(In1)
  Triggered Subsystem/1(Out1) -> Sum/1
  In1/1 -> Triggered Subsystem/Trigger
  Sum/1 -> Out1/1

== system hard_threshold_fixed_multichannel/check_refractory/Subsystem8/Time since last event  ==
  In1 : Inport
  Digital Clock : DigitalClock  SampleTime=1/32e3
  Sum : Sum  Inputs=|-+
  Triggered Subsystem : Subsystem  TreatAsAtomicUnit=on
  Out1 : Outport
  wires:
  Digital Clock/1 -> Sum/2, Triggered Subsystem/1(In1)
  Triggered Subsystem/1(Out1) -> Sum/1
  In1/1 -> Triggered Subsystem/Trigger
  Sum/1 -> Out1/1

== system hard_threshold_fixed_multichannel/check_refractory/Subsystem9/Time since last event  ==
  In1 : Inport
  Digital Clock : DigitalClock  SampleTime=1/32e3
  Sum : Sum  Inputs=|-+
  Triggered Subsystem : Subsystem  TreatAsAtomicUnit=on
  Out1 : Outport
  wires:
  Digital Clock/1 -> Sum/2, Triggered Subsystem/1(In1)
  Triggered Subsystem/1(Out1) -> Sum/1
  In1/1 -> Triggered Subsystem/Trigger
  Sum/1 -> Out1/1

== system hard_threshold_fixed_multichannel/check_refractory/Subsystem/Time since last event /Triggered Subsystem ==
  In1 : Inport
  Trigger : TriggerPort  VariantControl=Variant
  Out1 : Outport
  wires:
  In1/1 -> Out1/1

== system hard_threshold_fixed_multichannel/check_refractory/Subsystem1/Time since last event /Triggered Subsystem ==
  In1 : Inport
  Trigger : TriggerPort  VariantControl=Variant
  Out1 : Outport
  wires:
  In1/1 -> Out1/1

== system hard_threshold_fixed_multichannel/check_refractory/Subsystem10/Time since last event /Triggered Subsystem ==
  In1 : Inport
  Trigger : TriggerPort  VariantControl=Variant
  Out1 : Outport
  wires:
  In1/1 -> Out1/1

== system hard_threshold_fixed_multichannel/check_refractory/Subsystem11/Time since last event /Triggered Subsystem ==
  In1 : Inport
  Trigger : TriggerPort  VariantControl=Variant
  Out1 : Outport
  wires:
  In1/1 -> Out1/1

== system hard_threshold_fixed_multichannel/check_refractory/Subsystem12/Time since last event /Triggered Subsystem ==
  In1 : Inport
  Trigger : TriggerPort  VariantControl=Variant
  Out1 : Outport
  wires:
  In1/1 -> Out1/1

== system hard_threshold_fixed_multichannel/check_refractory/Subsystem13/Time since last event /Triggered Subsystem ==
  In1 : Inport
  Trigger : TriggerPort  VariantControl=Variant
  Out1 : Outport
  wires:
  In1/1 -> Out1/1

== system hard_threshold_fixed_multichannel/check_refractory/Subsystem14/Time since last event /Triggered Subsystem ==
  In1 : Inport
  Trigger : TriggerPort  VariantControl=Variant
  Out1 : Outport
  wires:
  In1/1 -> Out1/1

== system hard_threshold_fixed_multichannel/check_refractory/Subsystem15/Time since last event /Triggered Subsystem ==
  In1 : Inport
  Trigger : TriggerPort  VariantControl=Variant
  Out1 : Outport
  wires:
  In1/1 -> Out1/1

== system hard_threshold_fixed_multichannel/check_refractory/Subsystem16/Time since last event /Triggered Subsystem ==
  In1 : Inport
  Trigger : TriggerPort  VariantControl=Variant
  Out1 : Outport
  wires:
  In1/1 -> Out1/1

== system hard_threshold_fixed_multichannel/check_refractory/Subsystem17/Time since last event /Triggered Subsystem ==
  In1 : Inport
  Trigger : TriggerPort  VariantControl=Variant
  Out1 : Outport
  wires:
  In1/1 -> Out1/1

== system hard_threshold_fixed_multichannel/check_refractory/Subsystem18/Time since last event /Triggered Subsystem ==
  In1 : Inport
  Trigger : TriggerPort  VariantControl=Variant
  Out1 : Outport
  wires:
  In1/1 -> Out1/1

== system hard_threshold_fixed_multichannel/check_refractory/Subsystem19/Time since last event /Triggered Subsystem ==
  In1 : Inport
  Trigger : TriggerPort  VariantControl=Variant
  Out1 : Outport
  wires:
  In1/1 -> Out1/1

== system hard_threshold_fixed_multichannel/check_refractory/Subsystem2/Time since last event /Triggered Subsystem ==
  In1 : Inport
  Trigger : TriggerPort  VariantControl=Variant
  Out1 : Outport
  wires:
  In1/1 -> Out1/1

== system hard_threshold_fixed_multichannel/check_refractory/Subsystem20/Time since last event /Triggered Subsystem ==
  In1 : Inport
  Trigger : TriggerPort  VariantControl=Variant
  Out1 : Outport
  wires:
  In1/1 -> Out1/1

== system hard_threshold_fixed_multichannel/check_refractory/Subsystem21/Time since last event /Triggered Subsystem ==
  In1 : Inport
  Trigger : TriggerPort  VariantControl=Variant
  Out1 : Outport
  wires:
  In1/1 -> Out1/1

== system hard_threshold_fixed_multichannel/check_refractory/Subsystem22/Time since last event /Triggered Subsystem ==
  In1 : Inport
  Trigger : TriggerPort  VariantControl=Variant
  Out1 : Outport
  wires:
  In1/1 -> Out1/1

== system hard_threshold_fixed_multichannel/check_refractory/Subsystem23/Time since last event /Triggered Subsystem ==
  In1 : Inport
  Trigger : TriggerPort  VariantControl=Variant
  Out1 : Outport
  wires:
  In1/1 -> Out1/1

== system hard_threshold_fixed_multichannel/check_refractory/Subsystem24/Time since last event /Triggered Subsystem ==
  In1 : Inport
  Trigger : TriggerPort  VariantControl=Variant
  Out1 : Outport
  wires:
  In1/1 -> Out1/1

== system hard_threshold_fixed_multichannel/check_refractory/Subsystem25/Time since last event /Triggered Subsystem ==
  In1 : Inport
  Trigger : TriggerPort  VariantControl=Variant
  Out1 : Outport
  wires:
  In1/1 -> Out1/1

== system hard_threshold_fixed_multichannel/check_refractory/Subsystem26/Time since last event /Triggered Subsystem ==
  In1 : Inport
  Trigger : TriggerPort  VariantControl=Variant
  Out1 : Outport
  wires:
  In1/1 -> Out1/1

== system hard_threshold_fixed_multichannel/check_refractory/Subsystem27/Time since last event /Triggered Subsystem ==
  In1 : Inport
  Trigger : TriggerPort  VariantControl=Variant
  Out1 : Outport
  wires:
  In1/1 -> Out1/1

== system hard_threshold_fixed_multichannel/check_refractory/Subsystem28/Time since last event /Triggered Subsystem ==
  In1 : Inport
  Trigger : TriggerPort  VariantControl=Variant
  Out1 : Outport
  wires:
  In1/1 -> Out1/1

== system hard_threshold_fixed_multichannel/check_refractory/Subsystem29/Time since last event /Triggered Subsystem ==
  In1 : Inport
  Trigger : TriggerPort  VariantControl=Variant
  Out1 : Outport
  wires:
  In1/1 -> Out1/1

== system hard_threshold_fixed_multichannel/check_refractory/Subsystem3/Time since last event /Triggered Subsystem ==
  In1 : Inport
  Trigger : TriggerPort  VariantControl=Variant
  Out1 : Outport
  wires:
  In1/1 -> Out1/1

== system hard_threshold_fixed_multichannel/check_refractory/Subsystem30/Time since last event /Triggered Subsystem ==
  In1 : Inport
  Trigger : TriggerPort  VariantControl=Variant
  Out1 : Outport
  wires:
  In1/1 -> Out1/1

== system hard_threshold_fixed_multichannel/check_refractory/Subsystem31/Time since last event /Triggered Subsystem ==
  In1 : Inport
  Trigger : TriggerPort  VariantControl=Variant
  Out1 : Outport
  wires:
  In1/1 -> Out1/1

== system hard_threshold_fixed_multichannel/check_refractory/Subsystem4/Time since last event /Triggered Subsystem ==
  In1 : Inport
  Trigger : TriggerPort  VariantControl=Variant
  Out1 : Outport
  wires:
  In1/1 -> Out1/1

== system hard_threshold_fixed_multichannel/check_refractory/Subsystem5/Time since last event /Triggered Subsystem ==
  In1 : Inport
  Trigger : TriggerPort  VariantControl=Variant
  Out1 : Outport
  wires:
  In1/1 -> Out1/1

== system hard_threshold_fixed_multichannel/check_refractory/Subsystem6/Time since last event /Triggered Subsystem ==
  In1 : Inport
  Trigger : TriggerPort  VariantControl=Variant
  Out1 : Outport
  wires:
  In1/1 -> Out1/1

== system hard_threshold_fixed_multichannel/check_refractory/Subsystem7/Time since last event /Triggered Subsystem ==
  In1 : Inport
  Trigger : TriggerPort  VariantControl=Variant
  Out1 : Outport
  wires:
  In1/1 -> Out1/1

== system hard_threshold_fixed_multichannel/check_refractory/Subsystem8/Time since last event /Triggered Subsystem ==
  In1 : Inport
  Trigger : TriggerPort  VariantControl=Variant
  Out1 : Outport
  wires:
  In1/1 -> Out1/1

== system hard_threshold_fixed_multichannel/check_refractory/Subsystem9/Time since last event /Triggered Subsystem ==
  In1 : Inport
  Trigger : TriggerPort  VariantControl=Variant
  Out1 : Outport
  wires:
  In1/1 -> Out1/1
